simulink library "fbw_library"  (R2020b)
settings: Solver=VariableStepAuto  StartTime=0.0  StopTime=10.0  RelTol=1e-3
settings Model: Creator=Andreas  LastModifiedBy=Andreas

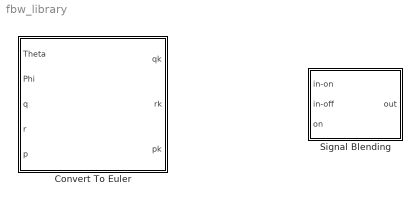
== system fbw_library ==
  Convert To Euler : MATLAB Function  TreatAsAtomicUnit=on
  Signal Blending : Subsystem
      mask Display:
      | port_label('input', 1, 'in_{on}', 'texmode', 'on')
      | port_label('input', 2, 'in_{off}', 'texmode', 'on')
      | port_label('input', 3, 'on', 'texmode', 'on')
      | 
      | port_label('output', 1, 'out', 'texmode', 'on')

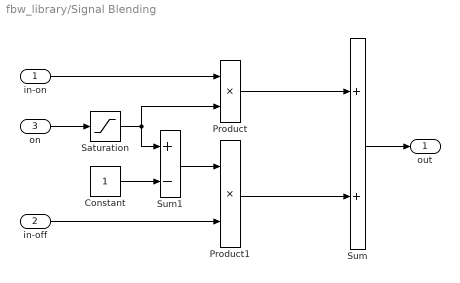
== system fbw_library/Signal Blending ==
  in-on : Inport
  in-off : Inport  Port=2
  on : Inport  Port=3
  Constant : Constant
  Product : Product
  Product1 : Product
  Saturation : Saturate  UpperLimit=1  LowerLimit=0
  Sum : Sum
  Sum1 : Sum  Inputs=+-
  out : Outport
  wires:
  Saturation/1 -> Sum1/1, Product/2
  in-off/1 -> Product1/2
  Constant/1 -> Sum1/2
  in-on/1 -> Product/1
  Sum1/1 -> Product1/1
  Sum/1 -> out/1
  Product1/1 -> Sum/2
  Product/1 -> Sum/1
  on/1 -> Saturation/1

== matlab function fbw_library/Convert To Euler ==
  data: Theta input; qk output; Phi input; q input; r input; p input; rk output; pk output
function [qk, rk, pk] = fbw_transform_to_euler(Theta, Phi, q, r, p)
  % read values
  Theta = deg2rad(Theta);
  Phi = deg2rad(Phi);

  % define transformation matrix
  transformation_matrix = [1, sin(Phi)*tan(Theta), cos(Phi)*tan(Theta); 0, cos(Phi), -sin(Phi); 0, sin(Phi)*sec(Theta), cos(Phi)*sec(Theta)];
  
  % define multiplication vector
  input = [p; q; r];

  % calculate result
  result = transformation_matrix * input;

  % assign results
  qk = result(2);
  rk = result(3);
  pk = result(1);
end
